simulink model "Simulation_estimetion_J"  (R2022b)
settings: Solver=VariableStepAuto  StartTime=0.0  StopTime=16.0  RelTol=1e-3
undefined symbols (not defined in the file or in its folder): motor, uc
libraries: fl_lib x13, nesl_utility x7, ee_lib x2, simulink x2
settings Model: Creator=berti  LastModifiedBy=berti
settings DataIOCC: SaveFormat=StructureWithTime

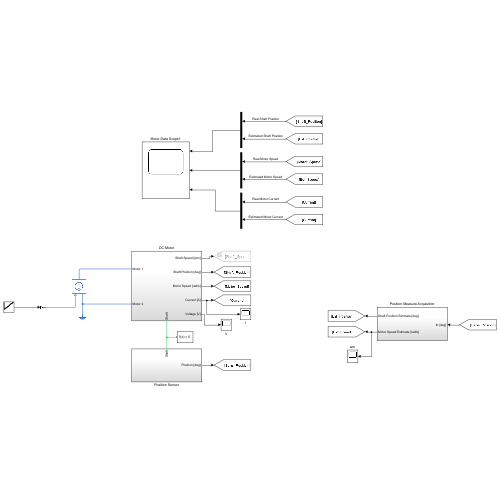
[thumbnail: Simulink's stored preview of the top-level diagram]
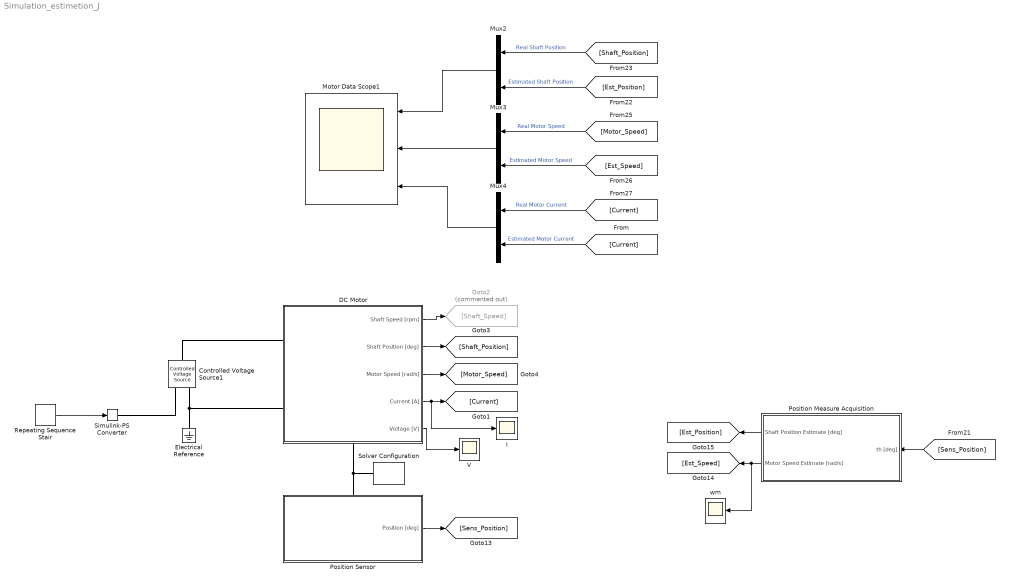
== system Simulation_estimetion_J ==
  Controlled Voltage Source1 : fl_lib/Electrical/Electrical Sources/Controlled Voltage Source
  DC Motor : Subsystem
      settings: PortSchema="{\"entries\":[{\"content\":{\"sides\":[{\"content\":{\"connectorIds\":[\"LConn1\",\"LConn2\"]},\"type\":\"ConnectorPlacement.EquallySpacedRectSide\",\"uuid\":\"6ab8a2ca-2e71-4c35-afcd-8b0bd2021176\"},{\"content\":{\"connectorIds\":[\"Out1\",\"Out2\",\"Out3\",\"Out4\",\"Out5\"],\"side\":\"RIGHT\"},\"type\":\"ConnectorPlacement.EquallySpacedRectSide\",\"uuid\":\"d3dfdd51-7397-4825-b175-78eac32e6d9d\"},{\"content\":{\"connectorIds\":[],\"side\":\"TOP\"},\"type\":\"ConnectorPlacement.EquallySpacedRectSide\",\"uuid\":\"a7cfaff2-0ae6-4fbb-a099-2a304565fee1\"},{\"content\":{\"connectorIds\":[\"RConn1\"],\"side\":\"BOTTOM\"},\"type\":\"ConnectorPlacement.EquallySpacedRectSide\",\"uuid\":\"a0639675-2e22-459b-8bb8-2c2f061728b4\"}]},\"type\":\"ConnectorPlacement.EquallySpacedConnector\",\"uuid\":\"c5b7cd6c-5a44-4892-a55d-8579e461572d\"}],\"packageUris\":[\"http://schema.mathworks.com/mf0/Connector/R2020b\"],\"version\":\"1.0\"}"
  Electrical Reference : fl_lib/Electrical/Electrical Elements/Electrical Reference
  Goto2 : Goto  Commented=on  GotoTag=Shaft_Speed
  I : Scope
  Motor Data Scope1 : Scope  NumInputPorts=3
  Mux2 : Mux  Inputs=2
  Mux3 : Mux  Inputs=2
  Mux4 : Mux  Inputs=2
  Position Measure Acquisition : Subsystem
  Position Sensor : Subsystem
      settings: PortSchema="{\"entries\":[{\"content\":{\"sides\":[{\"content\":{\"connectorIds\":[\"Out1\"]},\"type\":\"ConnectorPlacement.EquallySpacedRectSide\",\"uuid\":\"d36fe1c4-850a-4c75-8c52-3756b1598cdf\"},{\"content\":{\"connectorIds\":[],\"side\":\"RIGHT\"},\"type\":\"ConnectorPlacement.EquallySpacedRectSide\",\"uuid\":\"54a7c68c-1276-40fc-b30e-f6c2515c3006\"},{\"content\":{\"connectorIds\":[\"LConn1\"],\"side\":\"TOP\"},\"type\":\"ConnectorPlacement.EquallySpacedRectSide\",\"uuid\":\"1185fa4c-109a-4ade-aa58-e11090417f23\"}]},\"type\":\"ConnectorPlacement.EquallySpacedConnector\",\"uuid\":\"8f0159e8-c6cb-4893-a3e9-16e7311d52be\"}],\"packageUris\":[\"http://schema.mathworks.com/mf0/Connector/R2020b\"],\"version\":\"1.0\"}"
  Repeating Sequence Stair : simulink/Sources/Repeating Sequence Stair  OutValues=0.5 * [1 2 3 4 5 6 7 8].'  tsamp=t_delta1  OutMin=[]  OutMax=[]  OutDataTypeStr=double  OutputDataTypeScalingMode=double  OutDataType=fixdt(0,8)  ConRadixGroup=Best Precision: Vector-wise  OutScaling=2^-12
  Simulink-PS Converter : nesl_utility/Simulink-PS Converter  PhysicalDomain=network_engine_domain  SubClassName=ps_input  LeftPortType=input  RightPortType=output  PseudoPeriodic=off  Frequencies=[]  NoiseDistribution=none  NoiseParameters=[]  Unit=1  AffineConversion=off  FilteringAndDerivatives=provide  SimscapeFilterOrder=1  InputFilterTimeConstant=0.001  UdotUserProvided=0
  Solver Configuration : nesl_utility/Solver Configuration  PhysicalDomain=network_engine_domain  SubClassName=solver  LeftPortType=input  RightPortType=generic  Tones=[]  Harmonics=[]  SimulateNoise=off  Profile=off  UseLocalSampling=off  EnableSwitchedLinearOptims=on  FrequencyDomain=off  UseCCode=off  RelTol=0.001  AbsTol=0.001  MinStep=1e-09  ToWorkspace=off  RevertToSquareIcSolve=off  NumHomotopyIterations=100  PhasorMode=off  PhasorModeNumHarmonics=1  ConsistencySolver=NEWTON_XTOL_AFTER_FTOL  IndexReductionMethod=DerivativeReplacement  DoDC=off  ResidualTolerance=1e-09  ConsistencyTolSource=GLOBAL  ConsistencyAbsTol=0.001  ConsistencyRelTol=0.001  ConsistencyTolFactor=0.001  UseLocalSolver=off  LocalSolverChoice=NE_BACKWARD_EULER_ADVANCER  ResolveIndetEquations=on  FunctionEvalNumThread=1  LocalSolverSampleTime=0.001  DoFixedCost=off  MaxNonlinIter=3  MaxModeIter=2  ComputeImpulses=off  ImpulseIterations=2  LinearAlgebra=auto  LinearAlgebraNumThread=0  EquationFormulation=NE_TIME_EF  DelaysMemoryBudget=1024  AutomaticFiltering=on  FilteringTimeConstant=0.001  PartitionStorageMethod=AS_NEEDED  PartitionMemoryBudget=1024  PartitionMethod=ROBUST
  V : Scope
  wm : Scope
  wires:
  DC Motor/4(Current [A]) -> I/1, [Current]
  DC Motor/3(Motor Speed [rad/s]) -> [Motor_Speed]
  DC Motor/1(Shaft Speed [rpm]) -> Goto2/1
  Mux4/1 -> Motor Data Scope1/3
  Mux2/1 -> Motor Data Scope1/1
  DC Motor/2(Shaft Position [deg]) -> [Shaft_Position]
  Position Sensor/1(Position [deg]) -> [Sens_Position]
  [Est_Position] -> Mux2/2  "Estimated Shaft Position"
  [Est_Speed] -> Mux3/2  "Estimated Motor Speed"
  [Shaft_Position] -> Mux2/1  "Real Shaft Position"
  [Current] -> Mux4/1  "Real Motor Current"
  [Motor_Speed] -> Mux3/1  "Real Motor Speed"
  [Current] -> Mux4/2  "Estimated Motor Current"
  Mux3/1 -> Motor Data Scope1/2
  Position Measure Acquisition/1(Shaft Position Estimate [deg]) -> [Est_Position]
  Position Measure Acquisition/2(Motor Speed Estimate [rad/s]) -> wm/1, [Est_Speed]
  [Sens_Position] -> Position Measure Acquisition/1(th [deg])
  Repeating Sequence Stair/1 -> Simulink-PS Converter/1
  DC Motor/5(Voltage [V]) -> V/1
  connections:
  Position Sensor/LConn1 -- DC Motor/RConn1 -- Solver Configuration/RConn1
  DC Motor/LConn1 -- Controlled Voltage Source1/LConn1
  Controlled Voltage Source1/RConn2 -- DC Motor/LConn2 -- Electrical Reference/LConn1
  Simulink-PS Converter/RConn1 -- Controlled Voltage Source1/RConn1

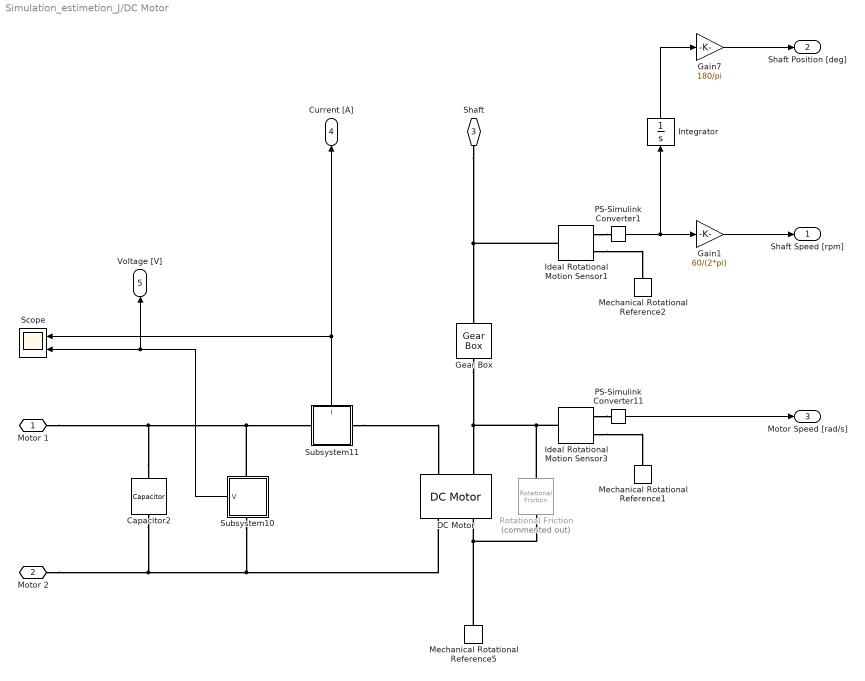
== system Simulation_estimetion_J/DC Motor ==
  Capacitor2 : fl_lib/Electrical/Electrical Elements/Capacitor  c=1e-6 F  r=1e-6 Ohm  g=0 1/Ohm  i_specify=off  i_priority=None  i=0 A  i_nominal_specify=off  i_nominal_unit=A  i_nominal_value=1  v_specify=off  v_priority=None  v=0 V  v_nominal_specify=off  v_nominal_unit=V  v_nominal_value=1  vc_specify=off  vc_priority=High  vc=0 V  vc_nominal_specify=off  vc_nominal_unit=V  vc_nominal_value=1
  DC Motor : ee_lib/Electromechanical/Brushed Motors/DC Motor  field_option=ee.enum.field_option.pm  Rf=100 Ohm  Lf=1 H  Laf=0.15 H  If0=0 A  parameterization=ee.enum.dcparam_option.torque_speed  Ra=motor.Ra Ohm  La=motor.La H  emf_or_torque=ee.enum.emf_or_torque.kv  Kv=motor.Kphi V/(rad/s)  Ki=6.876e-4 N*m/A  T_stall=motor.ts mN*m  w_max=motor.wmo rpm  w_rated=motor.wn rpm  P_rated=0.08 W  V_rated=motor.Vn V  lam_param=ee.enum.lam_param.current  i_noload=motor.Imo A  V_i_noload=motor.Vn V  J=motor.J kg*m^2  lam=motor.B N*m*s/rad  speed0=0 rpm  enable_fault_armature=simscape.enum.onoff.off  rev_faulted=1 / 3  G_faulted_armature=1e-5 S  fault_trigger_armature=ee.enum.faults.faultTrigger.temporal  t_fault_armature=1 s  max_permissible_current_armature=inf A  t_fail_on_current_armature=1 s  enable_fault_field=simscape.enum.onoff.off  G_faulted_field=1e-5 S  fault_trigger_field=ee.enum.faults.faultTrigger.temporal  t_fault_field=1 s  max_permissible_current_field=inf A  t_fail_on_current_field=1 s  fault_action=simscape.enum.assert.action.none  alpha=3.93e-3 1/K  Tmeas=25 degC  thermal_mass=100 J/K  initial_temperature=25 degC
  Gain1 : Gain  Gain=60/(2*pi)
  Gain7 : Gain  Gain=180/pi
  Gear Box : fl_lib/Mechanical/Mechanisms/Gear Box  ratio=motor.gearbox  t_in_specify=off  t_in_priority=None  t_in=0 N*m  t_in_nominal_specify=off  t_in_nominal_unit=N*m  t_in_nominal_value=1  t_out_specify=off  t_out_priority=None  t_out=0 N*m  t_out_nominal_specify=off  t_out_nominal_unit=N*m  t_out_nominal_value=1
  Ideal Rotational Motion Sensor1 : fl_lib/Mechanical/Mechanical Sensors/Ideal Rotational Motion Sensor  reference=foundation.enum.MeasurementReference.difference  acceleration_port=false  velocity_port=true  position_port=false  wrap_angle=false  offset=0 rad
      settings: InternalSimscapePortConfiguration="{\"Bottom\":[],\"Left\":[{\"id\":\"R\",\"label\":\"R\",\"type\":\"foundation.mechanical.rotational.rotational\"}],\"Right\":[{\"id\":\"C\",\"label\":\"C\",\"type\":\"foundation.mechanical.rotational.rotational\"},{\"id\":\"W\",\"label\":\"W\",\"type\":\"output\"}],\"Top\":[]}"
  Ideal Rotational Motion Sensor3 : fl_lib/Mechanical/Mechanical Sensors/Ideal Rotational Motion Sensor  reference=foundation.enum.MeasurementReference.difference  acceleration_port=false  velocity_port=true  position_port=false  wrap_angle=false  offset=0 rad
      settings: InternalSimscapePortConfiguration="{\"Bottom\":[],\"Left\":[{\"id\":\"R\",\"label\":\"R\",\"type\":\"foundation.mechanical.rotational.rotational\"}],\"Right\":[{\"id\":\"C\",\"label\":\"C\",\"type\":\"foundation.mechanical.rotational.rotational\"},{\"id\":\"W\",\"label\":\"W\",\"type\":\"output\"}],\"Top\":[]}"
  Integrator : Integrator
  Mechanical Rotational Reference1 : fl_lib/Mechanical/Rotational Elements/Mechanical Rotational Reference
  Mechanical Rotational Reference2 : fl_lib/Mechanical/Rotational Elements/Mechanical Rotational Reference
  Mechanical Rotational Reference5 : fl_lib/Mechanical/Rotational Elements/Mechanical Rotational Reference
  PS-Simulink Converter1 : nesl_utility/PS-Simulink Converter  PhysicalDomain=network_engine_domain  SubClassName=ps_output  LeftPortType=input  RightPortType=output  PseudoPeriodic=off  Frequencies=[]  VectorFormat=inherit  Unit=inherit  AffineConversion=off
  PS-Simulink Converter11 : nesl_utility/PS-Simulink Converter  PhysicalDomain=network_engine_domain  SubClassName=ps_output  LeftPortType=input  RightPortType=output  PseudoPeriodic=off  Frequencies=[]  VectorFormat=inherit  Unit=inherit  AffineConversion=off
  Rotational Friction : fl_lib/Mechanical/Rotational Elements/Rotational Friction  Commented=on  brkwy_trq=25 N*m  brkwy_vel=0.1 rad/s  Col_trq=20 N*m  visc_coef=0.001 N*m*s/rad  w_specify=off  w_priority=None  w=0 rad/s  w_nominal_specify=off  w_nominal_unit=rad/s  w_nominal_value=1  t_specify=off  t_priority=None  t=0 N*m  t_nominal_specify=off  t_nominal_unit=N*m  t_nominal_value=1
  Scope : Scope  NumInputPorts=2
  Subsystem10 : Subsystem
      settings: PortSchema="{\"entries\":[{\"content\":{\"sides\":[{\"content\":{\"connectorIds\":[]},\"type\":\"ConnectorPlacement.EquallySpacedRectSide\",\"uuid\":\"2573d3c3-03c4-452d-9dae-89011d1248da\"},{\"content\":{\"connectorIds\":[\"Out1\"],\"side\":\"RIGHT\"},\"type\":\"ConnectorPlacement.EquallySpacedRectSide\",\"uuid\":\"bbe9e370-74cc-46b8-9c24-075015e8eb10\"},{\"content\":{\"connectorIds\":[\"LConn1\"],\"side\":\"TOP\"},\"type\":\"ConnectorPlacement.EquallySpacedRectSide\",\"uuid\":\"b1ce1e52-8e1a-4765-9f85-bff289c8debb\"},{\"content\":{\"connectorIds\":[\"RConn1\"],\"side\":\"BOTTOM\"},\"type\":\"ConnectorPlacement.EquallySpacedRectSide\",\"uuid\":\"0695d450-f3c3-4287-93b9-efed01157391\"}]},\"type\":\"ConnectorPlacement.EquallySpacedConnector\",\"uuid\":\"9343d1eb-a2ec-4ec0-8fde-8976568d4d89\"}],\"packageUris\":[\"http://schema.mathworks.com/mf0/Connector/R2020b\"],\"version\":\"1.0\"}"
  Subsystem11 : Subsystem
      settings: PortSchema="{\"entries\":[{\"content\":{\"sides\":[{\"content\":{\"connectorIds\":[]},\"type\":\"ConnectorPlacement.EquallySpacedRectSide\",\"uuid\":\"2573d3c3-03c4-452d-9dae-89011d1248da\"},{\"content\":{\"connectorIds\":[\"Out1\"],\"side\":\"RIGHT\"},\"type\":\"ConnectorPlacement.EquallySpacedRectSide\",\"uuid\":\"bbe9e370-74cc-46b8-9c24-075015e8eb10\"},{\"content\":{\"connectorIds\":[\"LConn1\"],\"side\":\"TOP\"},\"type\":\"ConnectorPlacement.EquallySpacedRectSide\",\"uuid\":\"b1ce1e52-8e1a-4765-9f85-bff289c8debb\"},{\"content\":{\"connectorIds\":[\"RConn1\"],\"side\":\"BOTTOM\"},\"type\":\"ConnectorPlacement.EquallySpacedRectSide\",\"uuid\":\"0695d450-f3c3-4287-93b9-efed01157391\"}]},\"type\":\"ConnectorPlacement.EquallySpacedConnector\",\"uuid\":\"9343d1eb-a2ec-4ec0-8fde-8976568d4d89\"}],\"packageUris\":[\"http://schema.mathworks.com/mf0/Connector/R2020b\"],\"version\":\"1.0\"}"
  Motor 1 : PMIOPort  Side=Left
  Motor 2 : PMIOPort  Port=2  Side=Left
  Shaft : PMIOPort  Port=3  Side=Right
  Shaft Speed [rpm] : Outport
  Shaft Position [deg] : Outport  Port=2
  Motor Speed [rad/s] : Outport  Port=3
  Current [A] : Outport  Port=4
  Voltage [V] : Outport  Port=5
  wires:
  Subsystem11/1(I) -> Scope/1, Current [A]/1
  PS-Simulink Converter11/1 -> Motor Speed [rad/s]/1
  Gain1/1 -> Shaft Speed [rpm]/1
  PS-Simulink Converter1/1 -> Integrator/1, Gain1/1
  Integrator/1 -> Gain7/1
  Gain7/1 -> Shaft Position [deg]/1
  Subsystem10/1(V) -> Scope/2, Voltage [V]/1
  connections:
  Capacitor2/RConn1 -- Motor 2/RConn1 -- Subsystem10/RConn1 -- DC Motor/RConn1
  Capacitor2/LConn1 -- Subsystem10/LConn1 -- Subsystem11/LConn1 -- Motor 1/RConn1
  Ideal Rotational Motion Sensor3/LConn1 -- Rotational Friction/LConn1 -- DC Motor/LConn2 -- Gear Box/RConn1
  Mechanical Rotational Reference5/LConn1 -- Rotational Friction/RConn1 -- DC Motor/RConn2
  Ideal Rotational Motion Sensor3/RConn1 -- Mechanical Rotational Reference1/LConn1
  Ideal Rotational Motion Sensor3/RConn2 -- PS-Simulink Converter11/LConn1
  Ideal Rotational Motion Sensor1/RConn2 -- PS-Simulink Converter1/LConn1
  Ideal Rotational Motion Sensor1/RConn1 -- Mechanical Rotational Reference2/LConn1
  Ideal Rotational Motion Sensor1/LConn1 -- Gear Box/LConn1 -- Shaft/RConn1
  Subsystem11/RConn1 -- DC Motor/LConn1

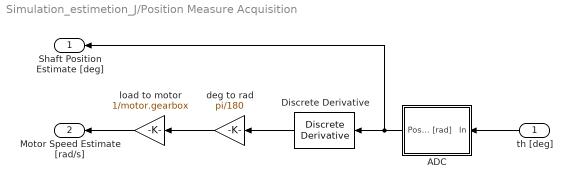
== system Simulation_estimetion_J/Position Measure Acquisition ==
  th [deg] : Inport
  ADC : Subsystem
  Discrete Derivative : simulink/Discrete/Discrete Derivative  gainval=1.0  ICPrevScaledInput=0.0  OutMin=[]  OutMax=[]  OutDataType=fixdt(1, 16)  OutScaling=2^-10  DoSatur=off
  deg to rad : Gain  Gain=pi/180
  load to motor : Gain  Gain=1/motor.gearbox
  Shaft Position Estimate [deg] : Outport
  Motor Speed Estimate [rad/s] : Outport  Port=2
  wires:
  th [deg]/1 -> ADC/1(In)
  ADC/1(Position Estimate [rad]) -> Discrete Derivative/1, Shaft Position Estimate [deg]/1
  Discrete Derivative/1 -> deg to rad/1
  load to motor/1 -> Motor Speed Estimate [rad/s]/1
  deg to rad/1 -> load to motor/1

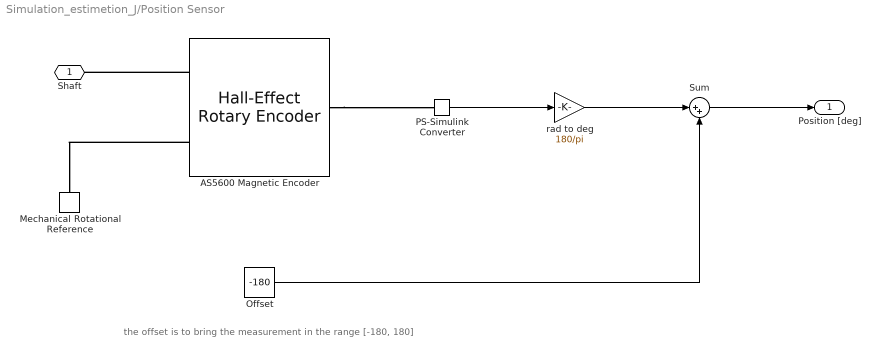
== system Simulation_estimetion_J/Position Sensor ==
  note: the offset is to bring the measurement in the range [-180, 180]
  AS5600 Magnetic Encoder : ee_lib/Sensors & Transducers/Hall-Effect Rotary Encoder  Ax=uc.pwr V  Ay=uc.pwr V  Vx0=0 V  Vy0=0 V  beta=0 deg  sensor_output=ee.enum.rotarysensors.output.decoded_ps  theta_specify=on  theta_priority=High  theta=180 deg  theta_nominal_specify=off  theta_nominal_unit=deg  theta_nominal_value=1
      settings: InternalSimscapePortConfiguration="{\"Bottom\":[],\"Left\":[{\"id\":\"R\",\"label\":\"R\",\"type\":\"foundation.mechanical.rotational.rotational\"},{\"id\":\"C\",\"label\":\"C\",\"type\":\"foundation.mechanical.rotational.rotational\"}],\"Right\":[{\"id\":\"A\",\"label\":\"Angle\",\"type\":\"output\"}],\"Top\":[]}"
  Mechanical Rotational Reference : fl_lib/Mechanical/Rotational Elements/Mechanical Rotational Reference
  Offset : Constant  Value=-180
  PS-Simulink Converter : nesl_utility/PS-Simulink Converter  PhysicalDomain=network_engine_domain  SubClassName=ps_output  LeftPortType=input  RightPortType=output  PseudoPeriodic=off  Frequencies=[]  VectorFormat=inherit  Unit=inherit  AffineConversion=off
  Sum : Sum  Inputs=|++
  rad to deg : Gain  Gain=180/pi
  Shaft : PMIOPort  Side=Left
  Position [deg] : Outport
  wires:
  rad to deg/1 -> Sum/1
  PS-Simulink Converter/1 -> rad to deg/1
  Sum/1 -> Position [deg]/1
  Offset/1 -> Sum/2
  connections:
  AS5600 Magnetic Encoder/LConn2 -- Mechanical Rotational Reference/LConn1
  AS5600 Magnetic Encoder/RConn1 -- PS-Simulink Converter/LConn1
  AS5600 Magnetic Encoder/LConn1 -- Shaft/RConn1

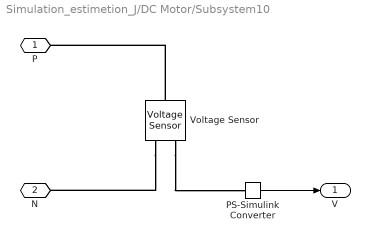
== system Simulation_estimetion_J/DC Motor/Subsystem10 ==
  PS-Simulink Converter : nesl_utility/PS-Simulink Converter  PhysicalDomain=network_engine_domain  SubClassName=ps_output  LeftPortType=input  RightPortType=output  PseudoPeriodic=off  Frequencies=[]  VectorFormat=inherit  Unit=inherit  AffineConversion=off
  Voltage Sensor : fl_lib/Electrical/Electrical Sensors/Voltage Sensor
  P : PMIOPort  Side=Left
  N : PMIOPort  Port=2  Side=Right
  V : Outport
  wires:
  PS-Simulink Converter/1 -> V/1
  connections:
  Voltage Sensor/RConn1 -- PS-Simulink Converter/LConn1
  Voltage Sensor/LConn1 -- P/RConn1
  Voltage Sensor/RConn2 -- N/RConn1

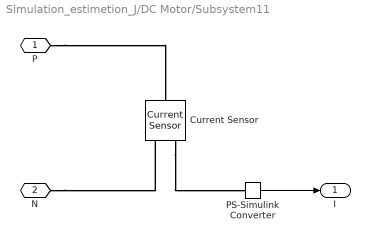
== system Simulation_estimetion_J/DC Motor/Subsystem11 ==
  Current Sensor : fl_lib/Electrical/Electrical Sensors/Current Sensor
  PS-Simulink Converter : nesl_utility/PS-Simulink Converter  PhysicalDomain=network_engine_domain  SubClassName=ps_output  LeftPortType=input  RightPortType=output  PseudoPeriodic=off  Frequencies=[]  VectorFormat=inherit  Unit=inherit  AffineConversion=off
  P : PMIOPort  Side=Left
  N : PMIOPort  Port=2  Side=Right
  I : Outport
  wires:
  PS-Simulink Converter/1 -> I/1
  connections:
  N/RConn1 -- Current Sensor/RConn2
  P/RConn1 -- Current Sensor/LConn1
  Current Sensor/RConn1 -- PS-Simulink Converter/LConn1

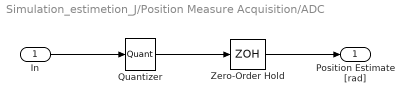
== system Simulation_estimetion_J/Position Measure Acquisition/ADC ==
  In : Inport
  Quantizer : Quantizer  QuantizationInterval=uc.adc_q
  Zero-Order Hold : ZeroOrderHold  SampleTime=uc.Ts
  Position Estimate [rad] : Outport
  wires:
  In/1 -> Quantizer/1
  Zero-Order Hold/1 -> Position Estimate [rad]/1
  Quantizer/1 -> Zero-Order Hold/1
